simulink model "stcex"  (Simulink 7.0)
settings: Solver=ode45  StartTime=0.0  StopTime=20.0  RelTol=1e-8
settings Model: Creator=Kailu  LastModifiedBy=Kailu  ExtModeTrigMode=oneshot  ExtModeArmWhenConnect=off
settings DataIOCC: LimitDataPoints=off
settings OptimizationCC: BlockReduction=off  BooleanDataType=off
settings DebuggingCC: SaveWithParameterizedLinksMsg=none  SignalResolutionControl=TryResolveAllWithWarning  SolverPrmCheckMsg=none  MultiTaskDSMMsg=warning  MultiTaskCondExecSysMsg=none  StrictBusMsg=None
settings HardwareCC: TargetUnknown=on
settings RTWCC: IncludeERTFirstTime=on

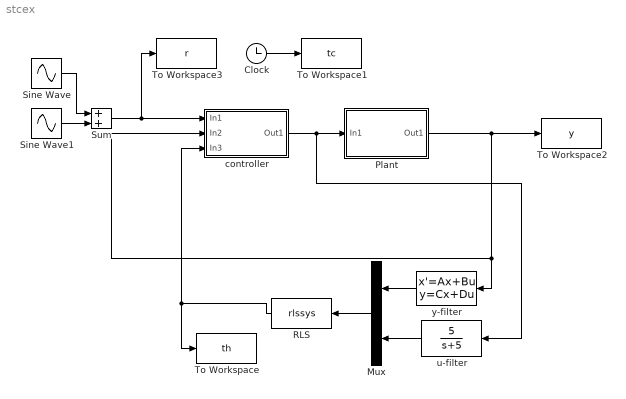
== system stcex ==
  Clock : Clock
      settings: Decimation=10
  Mux : Mux  Orientation=left  Inputs=2
  Plant : Subsystem
  RLS : S-Function  Orientation=left  FunctionName=rlssys  Parameters=[1;1],1000,2
  Sine Wave : Sin  SampleTime=0
  Sine Wave1 : Sin  Frequency=2  SampleTime=0
  Sum : Sum  SaturateOnIntegerOverflow=on  InputSameDT=on
  To Workspace : ToWorkspace  VariableName=th  SampleTime=0.01  SaveFormat=Array
  To Workspace1 : ToWorkspace  VariableName=tc  SampleTime=0.01  SaveFormat=Array
  To Workspace2 : ToWorkspace  VariableName=y  SampleTime=0.01  SaveFormat=Array
  To Workspace3 : ToWorkspace  VariableName=r  SampleTime=0.01  SaveFormat=Array
  controller : Subsystem
  u-filter : TransferFcn  Orientation=left  Numerator=[0 5]  Denominator=[1 5]
  y-filter : StateSpace  Orientation=left  A=-5  B=5  C=[-5;1]  D=[5;0]
  wires:
  Clock/1 -> To Workspace1/1
  Sine Wave/1 -> Sum/1
  Sine Wave1/1 -> Sum/2
  Plant/1(Out1) -> To Workspace2/1, controller/2(In2), y-filter/1
  Sum/1 -> controller/1(In1), To Workspace3/1
  controller/1(Out1) -> Plant/1(In1), u-filter/1
  u-filter/1 -> Mux/2
  Mux/1 -> RLS/1
  RLS/1 -> To Workspace/1, controller/3(In3)
  y-filter/1 -> Mux/1

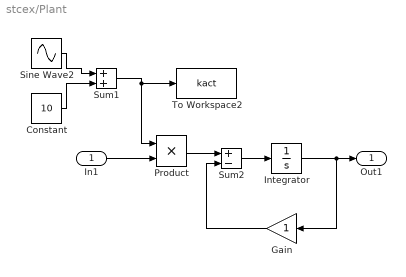
== system stcex/Plant ==
  In1 : Inport
  Constant : Constant  Value=10
  Gain : Gain  Orientation=left  SaturateOnIntegerOverflow=on
  Integrator : Integrator
  Product : Product  SaturateOnIntegerOverflow=on  RndMeth=Zero  InputSameDT=on
  Sine Wave2 : Sin  Frequency=0.5  SampleTime=0
  Sum1 : Sum  SaturateOnIntegerOverflow=on  InputSameDT=on
  Sum2 : Sum  Inputs=+-  SaturateOnIntegerOverflow=on  InputSameDT=on
  To Workspace2 : ToWorkspace  VariableName=kact  SampleTime=0.01  SaveFormat=Array
  Out1 : Outport
  wires:
  Sum2/1 -> Integrator/1
  Gain/1 -> Sum2/2
  Product/1 -> Sum2/1
  Sine Wave2/1 -> Sum1/1
  Constant/1 -> Sum1/2
  Integrator/1 -> Out1/1, Gain/1
  In1/1 -> Product/2
  Sum1/1 -> Product/1, To Workspace2/1

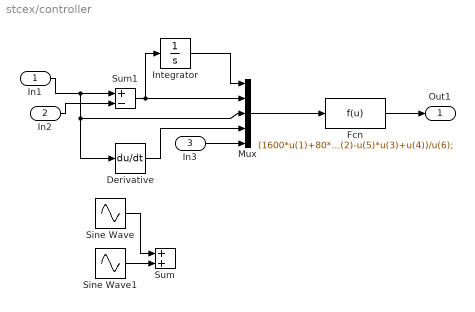
== system stcex/controller ==
  In1 : Inport
  In2 : Inport  Port=2
  In3 : Inport  Port=3
  Derivative : Derivative
  Fcn : Fcn  Expr=(1600*u(1)+80*u(2)-u(5)*u(3)+u(4))/u(6);
  Integrator : Integrator
  Mux : Mux  Inputs=5
  Sine Wave : Sin  Phase=pi/2  SampleTime=0
  Sine Wave1 : Sin  Amplitude=2  Frequency=2  Phase=pi/2  SampleTime=0
  Sum : Sum  SaturateOnIntegerOverflow=on  InputSameDT=on
  Sum1 : Sum  Inputs=+-  SaturateOnIntegerOverflow=on  InputSameDT=on
  Out1 : Outport
  wires:
  Integrator/1 -> Mux/1
  In2/1 -> Sum1/2
  In1/1 -> Sum1/1, Derivative/1, Mux/3
  Sum1/1 -> Mux/2, Integrator/1
  In3/1 -> Mux/5
  Mux/1 -> Fcn/1
  Fcn/1 -> Out1/1
  Sine Wave/1 -> Sum/1
  Sine Wave1/1 -> Sum/2
  Derivative/1 -> Mux/4
